simulink model "SMR_simplified_core"  (R2020a)
settings: Solver=VariableStepAuto  StartTime=0.0  StopTime=10.0  RelTol=1e-3
undefined symbols (not defined in the file): T_inlet
settings Model: Creator=marce  LastModifiedBy=tkdmc
settings DebuggingCC: AlgebraicLoopMsg=none

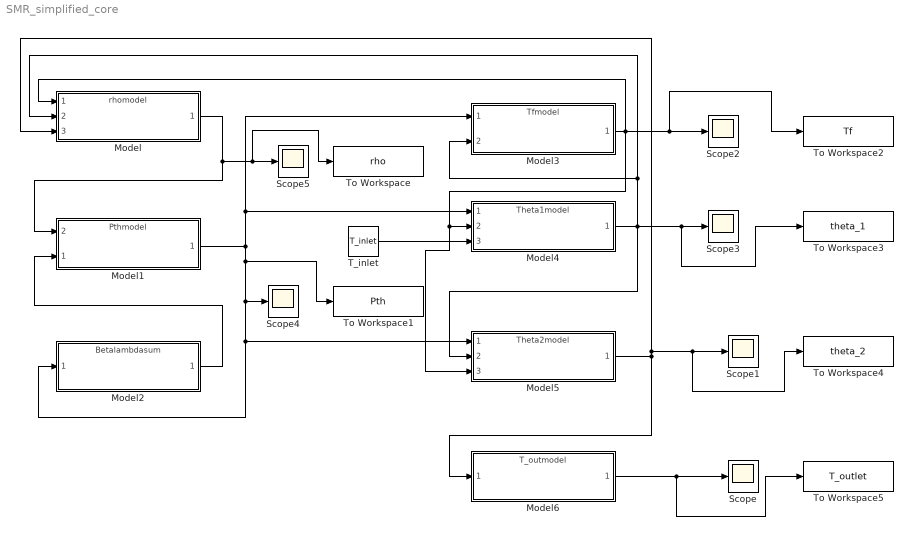
== system SMR_simplified_core ==
  Model : ModelReference  ModelNameDialog=rhomodel.slx  SimulationMode=Normal  ModelReferenceVersion=1.2
  Model1 : ModelReference  ModelNameDialog=Pthmodel.slx  SimulationMode=Normal  ModelReferenceVersion=1.2
      settings: PortSchema="{\"entries\":[{\"content\":{\"sides\":[{\"content\":{\"connectorIds\":[\"In2\",\"In1\"]},\"type\":\"ConnectorPlacement.EquallySpacedRectSide\",\"uuid\":\"e3224459-0710-4ae8-912c-ffc24afd85fc\"},{\"content\":{\"connectorIds\":[\"Out1\"],\"side\":\"RIGHT\"},\"type\":\"ConnectorPlacement.EquallySpacedRectSide\",\"uuid\":\"0843270c-201a-4a4e-9d3a-b74d02db8142\"},{\"content\":{\"connectorIds\":[],\"side\":\"TOP\"},\"type\":\"ConnectorPlacement.EquallySpacedRectSide\",\"uuid\":\"bb3babb0-06ba-491a-a610-e4cb28426240\"}]},\"type\":\"ConnectorPlacement.EquallySpacedConnector\",\"uuid\":\"0ed36f46-bfee-4649-aea5-de7db864205e\"}],\"packageUris\":[\"http://schema.mathworks.com/mf0/Connector/19700101\"],\"version\":\"1.0\"}"
  Model2 : ModelReference  ModelNameDialog=Betalambdasum.slx  SimulationMode=Normal  ModelReferenceVersion=1.5
  Model3 : ModelReference  ModelNameDialog=Tfmodel.slx  SimulationMode=Normal  ModelReferenceVersion=1.4
  Model4 : ModelReference  ModelNameDialog=Theta1model.slx  SimulationMode=Normal  ModelReferenceVersion=1.5
  Model5 : ModelReference  ModelNameDialog=Theta2model.slx  SimulationMode=Normal  ModelReferenceVersion=1.3
  Model6 : ModelReference  ModelNameDialog=T_outmodel.slx  SimulationMode=Normal  ModelReferenceVersion=1.3
  Scope{,1..5} (6 alike) : Scope
  T_inlet : Constant  Value=T_inlet
  To Workspace : ToWorkspace  VariableName=rho  SampleTime=-1
  To Workspace1 : ToWorkspace  VariableName=Pth  SampleTime=-1
  To Workspace2 : ToWorkspace  VariableName=Tf  SampleTime=-1
  To Workspace3 : ToWorkspace  VariableName=theta_1  SampleTime=-1
  To Workspace4 : ToWorkspace  VariableName=theta_2  SampleTime=-1
  To Workspace5 : ToWorkspace  VariableName=T_outlet  SampleTime=-1
  wires:
  Model2/1 -> Model1/1
  Model/1 -> Model1/2, To Workspace/1, Scope5/1
  Model1/1 -> To Workspace1/1, Scope4/1, Model5/1, Model2/1, Model4/1, Model3/1
  Model4/1 -> Model5/2, To Workspace3/1, Scope3/1, Model/2, Model3/2
  Model3/1 -> Model5/3, Model4/2, To Workspace2/1, Scope2/1, Model/1
  Model5/1 -> To Workspace4/1, Scope1/1, Model/3, Model6/1
  T_inlet/1 -> Model4/3
  Model6/1 -> To Workspace5/1, Scope/1
